simulink model "SimulinkQ19"  (R2016a)
settings: Solver=VariableStepAuto  StartTime=0.0  StopTime=500  RelTol=1e-3
settings Model: Creator=Lenovo  LastModifiedBy=Lenovo

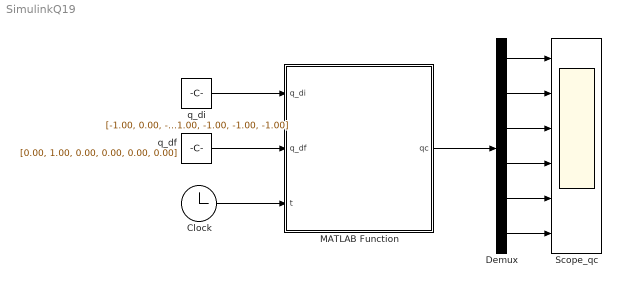
== system SimulinkQ19 ==
  Clock : Clock
  Demux : Demux  Outputs=6
  MATLAB Function : MATLAB Function  TreatAsAtomicUnit=on
  Scope_qc : Scope  NumInputPorts=6
  q_df : Constant  Value=[0.00, 1.00, 0.00, 0.00, 0.00, 0.00]
  q_di : Constant  Value=[-1.00, 0.00, -1.00, -1.00, -1.00, -1.00]
  wires:
  MATLAB Function/1(qc) -> Demux/1
  Demux/1 -> Scope_qc/1
  Demux/2 -> Scope_qc/2
  Demux/3 -> Scope_qc/3
  Demux/4 -> Scope_qc/4
  Demux/5 -> Scope_qc/5
  Demux/6 -> Scope_qc/6
  Clock/1 -> MATLAB Function/3(t)
  q_di/1 -> MATLAB Function/1(q_di)
  q_df/1 -> MATLAB Function/2(q_df)

== matlab function SimulinkQ19/MATLAB Function ==
  data: q_di input; qc output; q_df input; t input
function qc = GenTraj(q_di, q_df, t)
    tf = 500;
    D = q_df - q_di;
    r = 10*(t/tf)^3 -15*(t/tf)^4 + 6*(t/tf)^5;
    qc = q_di + r*D
end
